simulink model "SSnonLinearClosedLoop"  (Simulink 7.9)
settings: Solver=ode45  StartTime=0.0  StopTime=20  RelTol=1e-3
values from neighbouring files (symbols this model uses):
  Km = 25.1e-3    (= 0.0251)    [parameters.m]
settings Model: Creator=gdiazh  LastModifiedBy=root
settings OptimizationCC: InitFltsAndDblsToZero=on
settings DebuggingCC: FcnCallInpInsideContextMsg=Use local settings  StrictBusMsg=Warning
settings SFSimCC: SimParseCustomCode=off
settings GRTTargetCC: CombineOutputUpdateFcns=off  GRTInterface=on

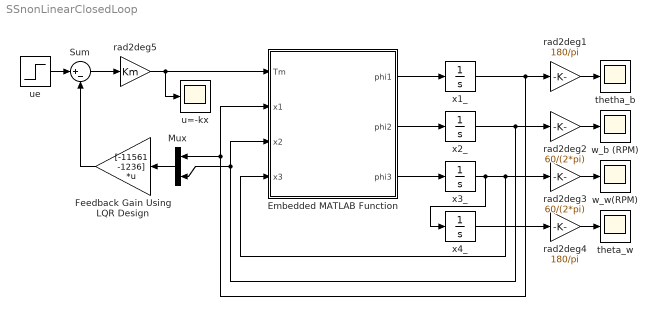
== system SSnonLinearClosedLoop ==
  Embedded MATLAB Function : MATLAB Function  TreatAsAtomicUnit=on
  Feedback Gain Using LQR Design : Gain  Gain="[-11561   -1236]"  Multiplication=Matrix(K*u) (u vector)
  Mux : Mux  Inputs=2
  Sum : Sum  Inputs=|+-
  rad2deg1 : Gain  Gain=180/pi  SaturateOnIntegerOverflow=on  OutDataTypeStr=Inherit: Same as input  ParamDataTypeStr=Inherit: Same as input
  rad2deg2 : Gain  Gain=60/(2*pi)  SaturateOnIntegerOverflow=on  OutDataTypeStr=Inherit: Same as input  ParamDataTypeStr=Inherit: Same as input
  rad2deg3 : Gain  Gain=60/(2*pi)  SaturateOnIntegerOverflow=on  OutDataTypeStr=Inherit: Same as input  ParamDataTypeStr=Inherit: Same as input
  rad2deg4 : Gain  Gain=180/pi  SaturateOnIntegerOverflow=on  OutDataTypeStr=Inherit: Same as input  ParamDataTypeStr=Inherit: Same as input
  rad2deg5 : Gain  Gain=Km  SaturateOnIntegerOverflow=on  OutDataTypeStr=Inherit: Same as input  ParamDataTypeStr=Inherit: Same as input
  theta_w : Scope
      settings: SaveName=angularVel
  thetha_b : Scope
      settings: TimeRange=20  YMin=0.0009375  YMax=0.0009445  SaveName=position
  u=-kx : Scope
      settings: YMin=1.38778e-17  YMax=0.5  SaveName=position1
  ue : Step  Time=0  After=0
  w_b (RPM) : Scope
      settings: TimeRange=20  YMin=-150  YMax=150  SaveName=theta
  w_w(RPM) : Scope
      settings: YMin=-1.725  YMax=-1.4  SaveName=linealVel
  x1_ : Integrator  InitialCondition=10*pi/180  UpperSaturationLimit=50  LowerSaturationLimit=-50
  x2_ : Integrator  InitialCondition=1  UpperSaturationLimit=2*pi  LowerSaturationLimit=0
  x3_ : Integrator  InitialCondition=1  UpperSaturationLimit=10  LowerSaturationLimit=-10
  x4_ : Integrator  UpperSaturationLimit=100  LowerSaturationLimit=-100
  wires:
  rad2deg4/1 -> theta_w/1
  rad2deg1/1 -> thetha_b/1
  rad2deg3/1 -> w_w(RPM)/1
  Embedded MATLAB Function/1(phi1) -> x1_/1
  Embedded MATLAB Function/2(phi2) -> x2_/1
  Embedded MATLAB Function/3(phi3) -> x3_/1
  x1_/1 -> rad2deg1/1, Embedded MATLAB Function/2(x1), Mux/1
  x2_/1 -> rad2deg2/1, Embedded MATLAB Function/3(x2), Mux/2
  x3_/1 -> x4_/1, rad2deg3/1, Embedded MATLAB Function/4(x3)
  x4_/1 -> rad2deg4/1
  rad2deg2/1 -> w_b (RPM)/1
  Mux/1 -> Feedback Gain Using LQR Design/1
  ue/1 -> Sum/1
  Sum/1 -> rad2deg5/1
  rad2deg5/1 -> u=-kx/1, Embedded MATLAB Function/1(Tm)
  Feedback Gain Using LQR Design/1 -> Sum/2

== matlab function Embedded MATLAB Function ==
  data: Tm input double; x1 input double; x2 input double; x3 input double; phi1 output double; phi2 output double; phi3 output double
function [phi1, phi2, phi3] = SSnonLinearModel(Tm, x1, x2, x3)
    %Valores de los parametros
    
    l  = 7e-2;      %[m]
    lb = 6e-2;      %[m]
    mb = 222.2e-3;  %[Kg]
    %mb = 419.0e-3;  %[Kg]
    mw = 22.9e-3;   %[Kg]
    %mw = 204e-3;   %[Kg]
    Ib = 1.62e-3;   %[Kg m^2]
    %Ib = 3.34e-3;   %[Kg m^2]
    Iw = 0.05e-3;   %[Kg m^2]
    %Iw = 0.57e-3;   %[Kg m^2]
    Cb = 1.02e-3;   %[Kg m^2 s^-1]
    Cw = 0.05e-3;   %[Kg m^2 s^-1]
    g  = 9.8;       %[m/s^2]
    
    phi1 = x2;
    
    num1 = (mb*lb+mw*l)*g*sin(x1)-Tm-Cb*x2+Cw*x3;
    phi2 = num1/(Ib+mw*l^2);
    
    num2 = (Iw+Ib+mw*l^2)*(Tm-Cw*x3);
    num3 = (mb*lb+mw*l)*g*sin(x1)-Cb*x2;
    phi3 = num2/(Iw*(Ib+mw*l^2))-num3/(Ib+mw*l^2);
end

%Ib=(222÷6)×(12÷100)²+(222)×(7÷100)²
